simulink model "opti_debug"  (R2023a)
settings: Solver=FixedStepAuto  StartTime=0.0  StopTime=mdl.rt  RelTol=1e-3
values from neighbouring files (symbols this model uses):
  archived_Eul_XYZ = rst_Eul_XYZ.signals.values    [s4_run.m]    (also in step4_run_v1.m)
  archived_p_raw = rst_p_raw.signals.values    [s4_run.m]    (also in step4_run_v1.m)
  ctr = make_ext_tor_observer(rsim, mdl, ctr)    [s1_setup.m]    (also in setup_controller_with_functions.m = make_controller(); step1_setup.m; step1_setup_v1.m)
  ctr2 = ctr    [s1_setup.m]    (also in step1_setup.m; step1_setup_v1.m)
  lut = gen_lut    [s1_setup.m]    (also in thrust2voltage_lut_20230809.mat = ; thrust2voltage_lut_20230829.mat = )
  mdl = make_model(mdl,rsim)    [s1_setup.m]    (also in setup_controller_with_functions.m = make_model(flight_time); step1_setup.m; step1_setup_v1.m = make_model(flight_time,rsim))
  rbt = make_robot    [s1_setup.m]    (also in setup_controller_with_functions.m = make_robot(); step1_setup.m; step1_setup_v1.m)
  rbt2 = rbt    [s1_setup.m]    (also in step1_setup.m; step1_setup_v1.m)
  rsim = make_robot_simulation()    [setup_controller_with_functions.m]    (also in step1_setup_v1.m = make_simulation(rbt,mdl,rsim))
  sen = make_sensor(mdl,rsim)    [s1_setup.m]
  som = make_somersault(mdl, rsim)    [s1_setup.m]    (also in step1_setup.m)
  Time = logsout.LiveStreamSignals.getElement('voltage').Values.Time    [old_step3_run_controller_v3.m]    (also in post_identify_actuation_response.m = yout(:,1); post_thrust_torque_coefficients.m = yout(:,1))
  traj = make_trajectory(ctr, mdl, rsim)    [s1_setup.m]    (also in step1_setup.m)
undefined symbols (not defined in the file or in its folder): DiscIntNeverNeededParam, Discrete, Standard_Devices, UDP_Protocol
libraries: simulink x27, dspfdesign x12, robotcorelib x7, sldrtlib x7, slrealtimeloglib x1, shared6dof x1, dspsrcs4 x1, uavutilslib x1, ctrlSharedLib x1, dspmathops x1
(part 2 of 4)

== system opti_debug/Motor thrust to voltage mapping/back mapping from sat volt to torque-thrust ==
  sat_voltages : Inport
  Demux5 : Demux
  Digital Filter Design2 : dspfdesign/Digital Filter Design  mwdsp_browser_bugfix_var=off
  Mux10 : Mux
  Nemo Bee 1 : Lookup_n-D  NumberOfTableDimensions=1  BreakpointsForDimension1=lut.v4  Table=lut.T4  InternalRulePriority=Speed  RndMeth=Simplest
  Nemo Bee 2 : Lookup_n-D  NumberOfTableDimensions=1  BreakpointsForDimension1=lut.v1  Table=lut.T1  InternalRulePriority=Speed  RndMeth=Simplest
  Nemo Bee 3 : Lookup_n-D  NumberOfTableDimensions=1  BreakpointsForDimension1=lut.v3  Table=lut.T3  InternalRulePriority=Speed  RndMeth=Simplest
  Nemo Bee 4 : Lookup_n-D  NumberOfTableDimensions=1  BreakpointsForDimension1=lut.v2  Table=lut.T2  InternalRulePriority=Speed  RndMeth=Simplest
  Saturation{6..9} (4 alike) : Saturate  UpperLimit=1000  LowerLimit=0
  Scope : Scope  NumInputPorts=2
  Scope1 : Scope  Commented=on
  power_distribution_1 : MATLAB Function  TreatAsAtomicUnit=on
  torque_thrust : Outport
  wires:
  Saturation9/1 -> Mux10/4
  Saturation7/1 -> Mux10/2
  Nemo Bee 1/1 -> Saturation9/1
  Demux5/3 -> Nemo Bee 3/1
  Demux5/1 -> Nemo Bee 2/1
  Nemo Bee 2/1 -> Saturation6/1
  Demux5/4 -> Nemo Bee 1/1
  Saturation8/1 -> Mux10/3
  Nemo Bee 4/1 -> Saturation7/1
  Saturation6/1 -> Mux10/1
  Nemo Bee 3/1 -> Saturation8/1
  Demux5/2 -> Nemo Bee 4/1
  sat_voltages/1 -> Demux5/1
  power_distribution_1/1(torque_thrust) -> Scope1/1, torque_thrust/1
  Mux10/1 -> Digital Filter Design2/1, Scope/1  "sat motor thrust (mgf)"
  Digital Filter Design2/1 -> power_distribution_1/1(motor_thrust), Scope/2  "filtered mtor thrust (mgf)"

== system opti_debug/Motor thrust to voltage mapping/voltage safety (no imag & NaN) ==
  In1 : Inport
  Complex to Real-Imag{,1..3} (4 alike) : ComplexToRealImag
  Delay{,1..3} (4 alike) : Delay  DelayLength=1
  Demux : Demux
  IsNaN{,1..3} (4 alike) : RelationalOperator  Operator=isNaN  OutDataTypeStr=boolean  RndMeth=Simplest  InputSameDT=off
  Mux : Mux
  Switch{1..3,17} (4 alike) : Switch  Criteria=u2 > Threshold  SaturateOnIntegerOverflow=off  InputSameDT=off
  Terminator{,1..3} (4 alike) : Terminator
  Output : Outport
  wires:
  In1/1 -> Demux/1
  IsNaN/1 -> Switch17/2
  Switch17/1 -> Delay1/1, Complex to Real-Imag/1
  Complex to Real-Imag/2 -> Terminator/1
  Demux/1 -> Switch17/3, IsNaN/1
  Complex to Real-Imag1/2 -> Terminator1/1
  Complex to Real-Imag1/1 -> Mux/2
  IsNaN1/1 -> Switch1/2
  Switch1/1 -> Delay/1, Complex to Real-Imag1/1
  Demux/2 -> Switch1/3, IsNaN1/1
  Complex to Real-Imag2/2 -> Terminator2/1
  Complex to Real-Imag2/1 -> Mux/3
  IsNaN2/1 -> Switch2/2
  Switch2/1 -> Delay2/1, Complex to Real-Imag2/1
  Demux/3 -> Switch2/3, IsNaN2/1
  Complex to Real-Imag3/2 -> Terminator3/1
  Complex to Real-Imag3/1 -> Mux/4
  IsNaN3/1 -> Switch3/2
  Demux/4 -> IsNaN3/1, Switch3/3
  Switch3/1 -> Delay3/1, Complex to Real-Imag3/1
  Mux/1 -> Output/1
  Complex to Real-Imag/1 -> Mux/1
  Delay/1 -> Switch1/1
  Delay1/1 -> Switch17/1
  Delay2/1 -> Switch2/1
  Delay3/1 -> Switch3/1

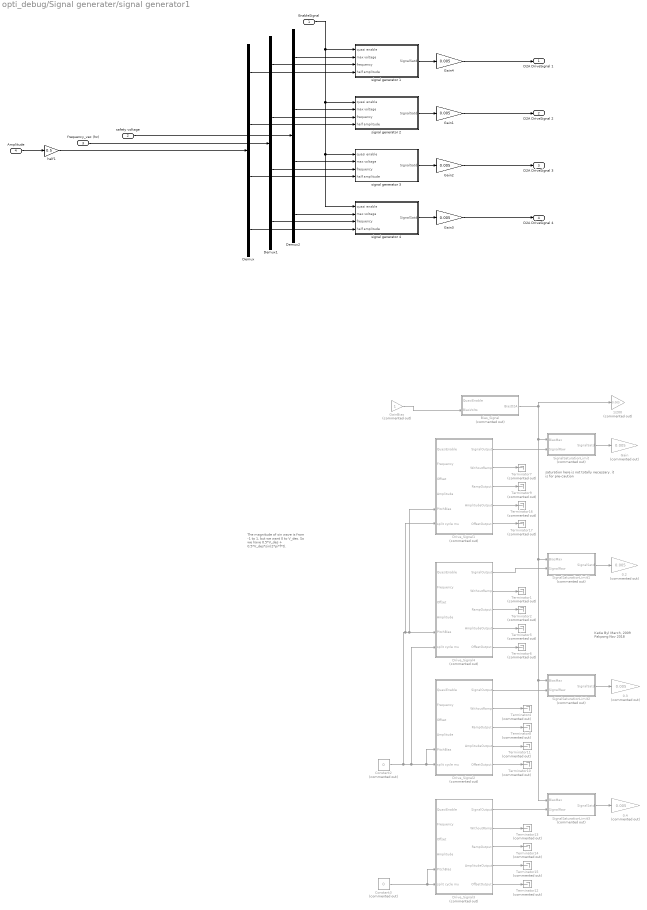
== system opti_debug/Signal generater/signal generator1 ==
  note: The magnitude of sin wave is from -1 to 1, but we want 0 to V_des. So we have 0.5*V_des + 0.5*V_des*sin(2*pi*f*t).
  note: Katie Byl
      | March, 2009
      |
      | Pakpong
      | Nov 2018
  note: saturation here is not totally necessary.
      | it is for pre-caution
  EnableSignal : Inport
  safety voltage : Inport  Port=2
  frequency_vec (hz) : Inport  Port=3
  Amplitude : Inport  Port=4
  0.2 : Gain  Commented=on  Gain=0.005
  0.3 : Gain  Commented=on  Gain=0.005
  0.4 : Gain  Commented=on  Gain=0.005
  1/200 : Gain  Commented=on  Gain=0.005
  Bias_Signal : Subsystem  Commented=on
  Constant2 : Constant  Commented=on  Value=0
  Constant3 : Constant  Commented=on  Value=0
  Demux : Demux
  Demux1 : Demux
  Demux2 : Demux
  Drive_Signal1 : Subsystem  Commented=on
  Drive_Signal2 : Subsystem  Commented=on
  Drive_Signal3 : Subsystem  Commented=on
  Drive_Signal4 : Subsystem  Commented=on
  Gain : Gain  Commented=on  Gain=0.005
  Gain{1..4} (4 alike) : Gain  Gain=0.005
  GainBias : Gain  Commented=on
  SignalSaturationLimit : Subsystem  Commented=on
  SignalSaturationLimit1 : Subsystem  Commented=on
  SignalSaturationLimit2 : Subsystem  Commented=on
  SignalSaturationLimit3 : Subsystem  Commented=on
  Terminator{1..2,4..17} (16 alike) : Terminator  Commented=on
  half1 : Gain  Gain=0.5
  signal generator 1 : Subsystem
  signal generator 2 : Subsystem
  signal generator 3 : Subsystem
  signal generator 4 : Subsystem
  D2A DriveSignal 1 : Outport
  D2A DriveSignal 2 : Outport  Port=2
  D2A DriveSignal 3 : Outport  Port=3
  D2A DriveSignal 4 : Outport  Port=4
  wires:
  Bias_Signal/1(BiasD2A) -> 1/200/1, SignalSaturationLimit3/1(BiasMax), SignalSaturationLimit2/1(BiasMax), SignalSaturationLimit1/1(BiasMax), SignalSaturationLimit/1(BiasMax)
  EnableSignal/1 -> signal generator 4/1(quasi enable), signal generator 3/1(quasi enable), signal generator 2/1(quasi enable), signal generator 1/1(quasi enable)
  SignalSaturationLimit/1(SignalSatd) -> Gain/1
  GainBias/1 -> Bias_Signal/2(BiasVolts)
  SignalSaturationLimit1/1(SignalSatd) -> 0.2/1
  Amplitude/1 -> half1/1
  Drive_Signal3/4(AmplitudeOutput) -> Terminator15/1
  Drive_Signal3/2(WithoutRamp) -> Terminator13/1
  Drive_Signal3/3(RampOutput) -> Terminator14/1
  Drive_Signal3/5(OffsetOutput) -> Terminator12/1
  Drive_Signal2/3(RampOutput) -> Terminator8/1
  Drive_Signal2/4(AmplitudeOutput) -> Terminator11/1
  Drive_Signal3/1(SignalOutput) -> SignalSaturationLimit3/2(SignalRaw)
  Drive_Signal2/5(OffsetOutput) -> Terminator10/1
  Drive_Signal2/2(WithoutRamp) -> Terminator4/1
  Demux/3 -> signal generator 3/4(half amplitude)
  Demux/4 -> signal generator 4/4(half amplitude)
  Constant2/1 -> Drive_Signal1/6(split cycle mu), Drive_Signal1/5(PitchBias), Drive_Signal4/5(PitchBias), Drive_Signal4/6(split cycle mu), Drive_Signal2/5(PitchBias), Drive_Signal2/6(split cycle mu)
  Constant3/1 -> Drive_Signal3/5(PitchBias), Drive_Signal3/6(split cycle mu)
  SignalSaturationLimit2/1(SignalSatd) -> 0.3/1
  SignalSaturationLimit3/1(SignalSatd) -> 0.4/1
  Drive_Signal2/1(SignalOutput) -> SignalSaturationLimit2/2(SignalRaw)
  half1/1 -> Demux/1
  frequency_vec (hz)/1 -> Demux1/1
  Demux1/1 -> signal generator 1/3(frequency)
  Demux1/2 -> signal generator 2/3(frequency)
  Demux1/3 -> signal generator 3/3(frequency)
  Demux1/4 -> signal generator 4/3(frequency)
  Drive_Signal4/1(SignalOutput) -> SignalSaturationLimit1/2(SignalRaw)
  Drive_Signal4/2(WithoutRamp) -> Terminator1/1
  Drive_Signal4/3(RampOutput) -> Terminator2/1
  Drive_Signal4/4(AmplitudeOutput) -> Terminator5/1
  Drive_Signal4/5(OffsetOutput) -> Terminator6/1
  Drive_Signal1/4(AmplitudeOutput) -> Terminator16/1
  Drive_Signal1/1(SignalOutput) -> SignalSaturationLimit/2(SignalRaw)
  Drive_Signal1/2(WithoutRamp) -> Terminator7/1
  Drive_Signal1/5(OffsetOutput) -> Terminator17/1
  Drive_Signal1/3(RampOutput) -> Terminator9/1
  Demux/1 -> signal generator 1/4(half amplitude)
  Demux/2 -> signal generator 2/4(half amplitude)
  signal generator 2/1(SignalSatd) -> Gain1/1
  signal generator 3/1(SignalSatd) -> Gain2/1
  signal generator 4/1(SignalSatd) -> Gain3/1
  signal generator 1/1(SignalSatd) -> Gain4/1
  Gain3/1 -> D2A DriveSignal 4/1
  Gain2/1 -> D2A DriveSignal 3/1
  Gain1/1 -> D2A DriveSignal 2/1
  Gain4/1 -> D2A DriveSignal 1/1
  safety voltage/1 -> Demux2/1
  Demux2/1 -> signal generator 1/2(max voltage)
  Demux2/2 -> signal generator 2/2(max voltage)
  Demux2/3 -> signal generator 3/2(max voltage)
  Demux2/4 -> signal generator 4/2(max voltage)

== system opti_debug/Signal generater/signal safety (no imag & NaN) ==
  In1 : Inport
  Complex to Real-Imag{,1..3} (4 alike) : ComplexToRealImag
  Constant{,1..3} (4 alike) : Constant  Value=0
  Demux : Demux
  IsNaN{,1..3} (4 alike) : RelationalOperator  Operator=isNaN  OutDataTypeStr=boolean  RndMeth=Simplest  InputSameDT=off
  Mux : Mux
  Switch{1..3,17} (4 alike) : Switch  Criteria=u2 > Threshold  SaturateOnIntegerOverflow=off  InputSameDT=off
  Terminator{,1..3} (4 alike) : Terminator
  Output : Outport
  wires:
  In1/1 -> Demux/1
  IsNaN/1 -> Switch17/2
  Constant/1 -> Switch17/1
  Switch17/1 -> Complex to Real-Imag/1
  Complex to Real-Imag/2 -> Terminator/1
  Demux/1 -> Switch17/3, IsNaN/1
  Complex to Real-Imag1/2 -> Terminator1/1
  Complex to Real-Imag1/1 -> Mux/2
  IsNaN1/1 -> Switch1/2
  Switch1/1 -> Complex to Real-Imag1/1
  Demux/2 -> Switch1/3, IsNaN1/1
  Constant1/1 -> Switch1/1
  Complex to Real-Imag2/2 -> Terminator2/1
  Complex to Real-Imag2/1 -> Mux/3
  IsNaN2/1 -> Switch2/2
  Switch2/1 -> Complex to Real-Imag2/1
  Demux/3 -> Switch2/3, IsNaN2/1
  Constant2/1 -> Switch2/1
  Complex to Real-Imag3/2 -> Terminator3/1
  Complex to Real-Imag3/1 -> Mux/4
  IsNaN3/1 -> Switch3/2
  Demux/4 -> IsNaN3/1, Switch3/3
  Switch3/1 -> Complex to Real-Imag3/1
  Constant3/1 -> Switch3/1
  Mux/1 -> Output/1
  Complex to Real-Imag/1 -> Mux/1

== system opti_debug/State filters/Acc through derivative ==
  Vicon_p_dot : Inport
  sim_p_dot : Inport  Port=2
  data ready : Inport  Port=3
  Add2 : Sum  Inputs=+-
  Constant3 : Constant  Value=rsim.en
  Delay1 : Delay  DelayLength=1  InitialCondition=zeros(3,1)
  Gain1 : Gain  Gain=400
  Subsystem1 : Subsystem
  Switch2 : Switch  Criteria=u2 > Threshold  SaturateOnIntegerOverflow=off  InputSameDT=off
  p_dotdot : Outport
  wires:
  Subsystem1/1(p_dotdot) -> Switch2/3
  sim_p_dot/1 -> Delay1/1, Add2/1
  Add2/1 -> Gain1/1
  Constant3/1 -> Switch2/2
  Delay1/1 -> Add2/2
  Vicon_p_dot/1 -> Subsystem1/1(p_dot)
  Switch2/1 -> p_dotdot/1  "p_dotdot"
  Gain1/1 -> Switch2/1
  data ready/1 -> Subsystem1/2(data ready)

== system opti_debug/State filters/IMU orientation ==
  sensor_Eul_XYZ : Inport
  Digital Filter Design1 : dspfdesign/Digital Filter Design  mwdsp_browser_bugfix_var=off
  Reshape2 : Reshape
  Subsystem2 : Subsystem
  Sensor_EulXYZ : Outport
  sensor_raw_omega : Outport  Port=2
  sensor_filt_omega : Outport  Port=3
  wires:
  sensor_Eul_XYZ/1 -> Subsystem2/1(euler_angles), Reshape2/1
  Digital Filter Design1/1 -> sensor_filt_omega/1  "sensor_filt_omega"
  Subsystem2/1(Omega) -> sensor_raw_omega/1, Digital Filter Design1/1  "sensor_raw_omega"
  Reshape2/1 -> Sensor_EulXYZ/1  "sensor_EulXYZ"

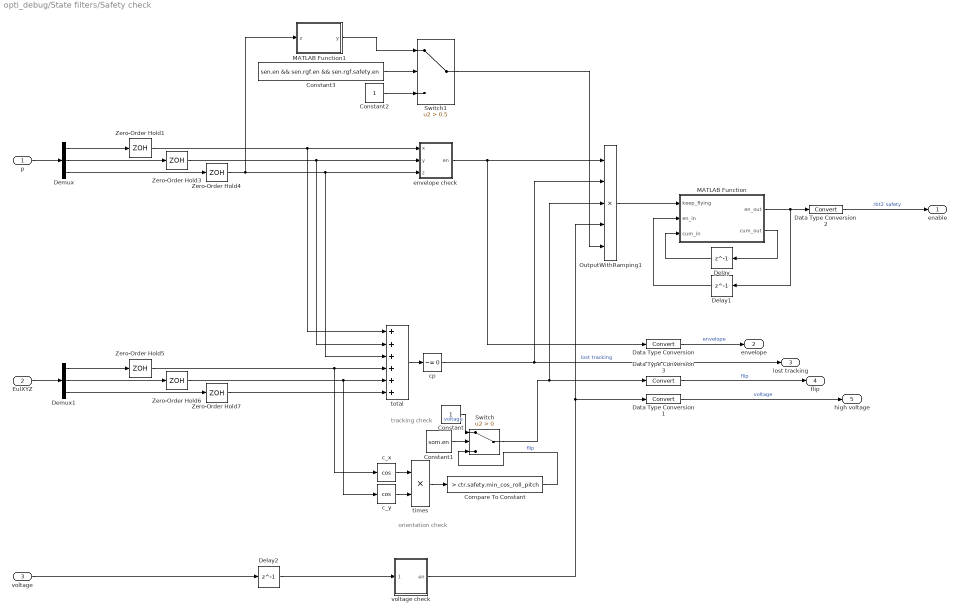
== system opti_debug/State filters/Safety check ==
  note: tracking check
  note: orientation check
  p : Inport
  EulXYZ : Inport  Port=2
  voltage : Inport  Port=3
  Compare To Constant : simulink/Logic and Bit Operations/Compare To Constant  relop=>  const=ctr.safety.min_cos_roll_pitch  OutDataTypeStr=uint8
  Constant : Constant
  Constant1 : Constant  Value=som.en
  Constant2 : Constant
  Constant3 : Constant  Value=sen.en && sen.rgf.en && sen.rgf.safety.en
  Data Type Conversion{,1..3} (4 alike) : DataTypeConversion  SaturateOnIntegerOverflow=off  RndMeth=Floor
  Delay : Delay  DelayLength=1
  Delay1 : Delay  DelayLength=1  InitialCondition=1
  Delay2 : Delay  DelayLength=1  InitialCondition=zeros(4,1)
  Demux : Demux  Outputs=3
  Demux1 : Demux  Outputs=3
  MATLAB Function : MATLAB Function  TreatAsAtomicUnit=on  SystemSampleTime=mdl.T
  MATLAB Function1 : MATLAB Function  TreatAsAtomicUnit=on
  OutputWithRamping1 : Product  Inputs=5  RndMeth=Zero
  Switch : Switch  Criteria=u2 > Threshold  SaturateOnIntegerOverflow=off  InputSameDT=off
  Switch1 : Switch  Criteria=u2 > Threshold  Threshold=0.5  SaturateOnIntegerOverflow=off  InputSameDT=off
  Zero-Order Hold{1,3..7} (6 alike) : ZeroOrderHold  SampleTime=mdl.T
  c_x : Trigonometry  Operator=cos
  c_y : Trigonometry  Operator=cos
  cp : simulink/Logic and Bit Operations/Compare To Zero  relop=~=  OutDataTypeStr=uint8
  envelope check : MATLAB Function  TreatAsAtomicUnit=on
  times : Product  RndMeth=Zero
  total : Sum  Inputs=++++++
  voltage check : MATLAB Function  TreatAsAtomicUnit=on
  enable : Outport
  envelope : Outport  Port=2
  lost tracking : Outport  Port=3
  flip : Outport  Port=4
  high voltage : Outport  Port=5
  wires:
  Zero-Order Hold3/1 -> envelope check/2(y), total/2
  cp/1 -> lost tracking/1, OutputWithRamping1/2  "lost tracking"
  Demux/3 -> Zero-Order Hold4/1
  times/1 -> Compare To Constant/1
  envelope check/1(en) -> Data Type Conversion/1, OutputWithRamping1/1
  Zero-Order Hold1/1 -> total/1, envelope check/1(x)
  Demux/2 -> Zero-Order Hold3/1
  OutputWithRamping1/1 -> MATLAB Function/1(keep_flying)
  Zero-Order Hold4/1 -> MATLAB Function1/1(z), total/3, envelope check/3(z)
  Demux1/2 -> Zero-Order Hold6/1
  MATLAB Function/2(cum_out) -> Delay/1
  Delay1/1 -> MATLAB Function/2(en_in)
  Data Type Conversion1/1 -> high voltage/1  "voltage"
  Data Type Conversion/1 -> envelope/1  "envelope"
  Delay2/1 -> voltage check/1(voltage)
  Switch/1 -> OutputWithRamping1/3, Data Type Conversion3/1
  total/1 -> cp/1
  Zero-Order Hold7/1 -> total/6
  Zero-Order Hold6/1 -> total/5, c_y/1
  voltage/1 -> Delay2/1
  Compare To Constant/1 -> Switch/3  "flip"
  MATLAB Function/1(en_out) -> Delay1/1, Data Type Conversion2/1
  Data Type Conversion2/1 -> enable/1  "rbt2 safety"
  Data Type Conversion3/1 -> flip/1  "flip"
  Constant1/1 -> Switch/2
  c_y/1 -> times/2
  Demux1/3 -> Zero-Order Hold7/1
  Delay/1 -> MATLAB Function/3(cum_in)
  voltage check/1(en) -> OutputWithRamping1/4, Data Type Conversion1/1
  Constant/1 -> Switch/1  "voltage"
  c_x/1 -> times/1
  Zero-Order Hold5/1 -> total/4, c_x/1
  p/1 -> Demux/1
  Demux/1 -> Zero-Order Hold1/1
  EulXYZ/1 -> Demux1/1
  Demux1/1 -> Zero-Order Hold5/1
  Constant2/1 -> Switch1/3
  Constant3/1 -> Switch1/2
  MATLAB Function1/1(y) -> Switch1/1
  Switch1/1 -> OutputWithRamping1/5

== system opti_debug/State filters/Velocity through derivative ==
  Vicon_p : Inport
  data ready : Inport  Port=2
  Add1 : Sum  Inputs=+-
  Constant2 : Constant  Value=rsim.en
  Delay : Delay  DelayLength=1  InitialCondition=zeros(3,1)
  Gain : Gain  Gain=400
  Subsystem4 : Subsystem
  Switch1 : Switch  Criteria=u2 > Threshold  SaturateOnIntegerOverflow=off  InputSameDT=off
  Vicon_p_dot : Outport
  sim_p_dot : Outport  Port=2
  wires:
  Delay/1 -> Add1/2
  Subsystem4/1(p dot) -> Switch1/3
  Vicon_p/1 -> Subsystem4/1(In1), Delay/1, Add1/1
  Constant2/1 -> Switch1/2
  Add1/1 -> Gain/1
  Switch1/1 -> Vicon_p_dot/1  "Vicon_p_dot"
  data ready/1 -> Subsystem4/2(data ready)
  Gain/1 -> sim_p_dot/1, Switch1/1  "sim_p_dot"

== system opti_debug/State filters/Vicon orientation ==
  Eul XYZ : Inport
  data_ready : Inport  Port=2
  Digital Filter Design2 : dspfdesign/Digital Filter Design  mwdsp_browser_bugfix_var=off
  Reshape1 : Reshape
  Subsystem5 : Subsystem
  Terminator8 : Terminator
  Terminator9 : Terminator
  Vicon_EulXYZ : Outport
  Vicon_raw_omega : Outport  Port=2
  Vicon_filt_omega : Outport  Port=3
  wires:
  Eul XYZ/1 -> Reshape1/1, Subsystem5/1(euler_angles)
  Reshape1/1 -> Vicon_EulXYZ/1  "Vicon_EulXYZ"
  Subsystem5/2(Rdot) -> Terminator9/1
  Subsystem5/3(Omega) -> Vicon_raw_omega/1, Digital Filter Design2/1  "Vicon_raw_omega"
  Subsystem5/1(R) -> Terminator8/1
  Digital Filter Design2/1 -> Vicon_filt_omega/1  "Vicon_filt_omega"
  data_ready/1 -> Subsystem5/2(data ready)

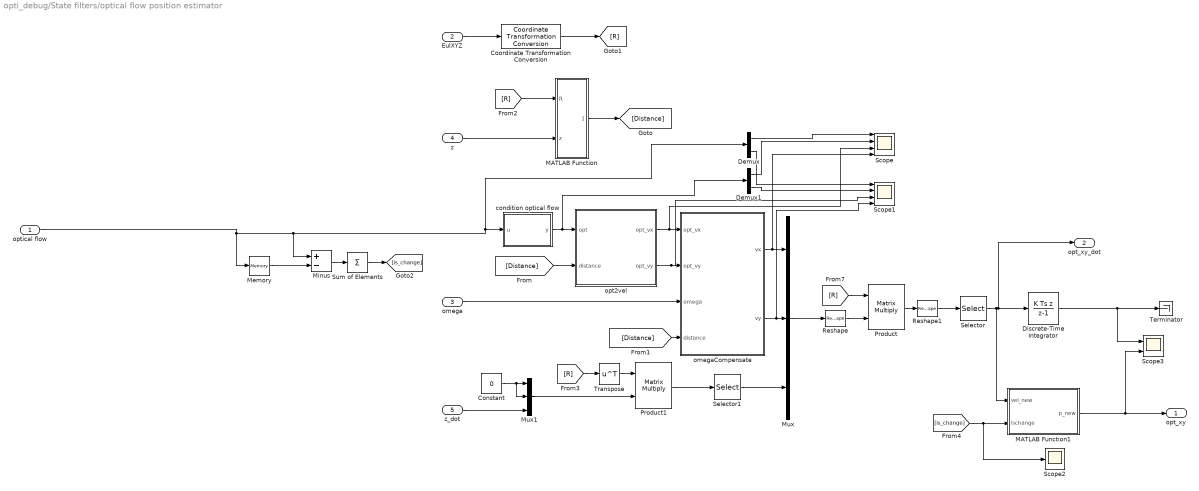
== system opti_debug/State filters/optical flow position estimator ==
  optical flow : Inport
  EulXYZ : Inport  Port=2
  omega : Inport  Port=3
  z : Inport  Port=4
  z_dot : Inport  Port=5
  Constant : Constant  Value=0
  Coordinate Transformation Conversion : robotcorelib/Coordinate Transformation Conversion  InputRepresentation=Euler Angles  InputEulerSequence=XYZ  ShowTrVecInputPort=on  OutputRepresentation=Rotation Matrix  OutputEulerSequence=ZYX  ShowTrVecOutputPort=on  SimulateUsing=Interpreted execution
  Demux : Demux  Outputs=2
  Demux1 : Demux  Outputs=2
  Discrete-Time Integrator : DiscreteIntegrator  IntegratorMethod=Integration: Backward Euler  InitialCondition=[0;0]  SampleTime=-1  ICPrevOutput=DiscIntNeverNeededParam  ICPrevScaledInput=DiscIntNeverNeededParam
  MATLAB Function : MATLAB Function  TreatAsAtomicUnit=on  SystemSampleTime=mdl.T_high
  MATLAB Function1 : MATLAB Function  TreatAsAtomicUnit=on
  Memory : Memory
  Minus : Sum  Inputs=+-
  Mux : Mux  Inputs=3
  Mux1 : Mux  Inputs=3
  Product : Product  Multiplication=Matrix(*)
  Product1 : Product  Multiplication=Matrix(*)
  Reshape : Reshape  OutputDimensionality=Column vector (2-D)
  Reshape1 : Reshape
  Scope : Scope  NumInputPorts=4
  Scope1 : Scope  NumInputPorts=4
  Scope2 : Scope
  Scope3 : Scope  NumInputPorts=2
  Selector : Selector  InputPortWidth=3  IndexOptions=Index vector (dialog)  Indices=[1 2 ]  OutputSizes=1
  Selector1 : Selector  InputPortWidth=3  IndexOptions=Index vector (dialog)  Indices=[3 ]  OutputSizes=1
  Sum of Elements : Sum  Inputs=+
  Terminator : Terminator
  Transpose : Math  Operator=transpose
  condition optical flow : MATLAB Function  TreatAsAtomicUnit=on
  omegaCompensate : MATLAB Function  TreatAsAtomicUnit=on
  opt2vel : MATLAB Function  TreatAsAtomicUnit=on
  opt_xy : Outport
  opt_xy_dot : Outport  Port=2
  wires:
  EulXYZ/1 -> Coordinate Transformation Conversion/1
  z/1 -> MATLAB Function/2(z)
  MATLAB Function/1(distance) -> [Distance]
  [Distance] -> opt2vel/2(distance)
  opt2vel/1(opt_vx) -> Scope/3, omegaCompensate/1(opt_vx)
  opt2vel/2(opt_vy) -> Scope1/3, omegaCompensate/2(opt_vy)
  [Distance] -> omegaCompensate/4(distance)
  omega/1 -> omegaCompensate/3(omega)
  Coordinate Transformation Conversion/1 -> [R]
  [R] -> MATLAB Function/1(R)
  [R] -> Product/1
  Reshape/1 -> Product/2
  Mux/1 -> Reshape/1
  omegaCompensate/1(vx) -> Scope/4, Mux/1
  omegaCompensate/2(vy) -> Scope1/4, Mux/2
  Product/1 -> Reshape1/1
  Reshape1/1 -> Selector/1
  [R] -> Transpose/1
  Transpose/1 -> Product1/1
  Product1/1 -> Selector1/1
  Constant/1 -> Mux1/2, Mux1/1
  z_dot/1 -> Mux1/3
  Mux1/1 -> Product1/2
  Selector1/1 -> Mux/3
  Selector/1 -> MATLAB Function1/1(vel_new), opt_xy_dot/1, Discrete-Time Integrator/1
  condition optical flow/1(y) -> Demux1/1, opt2vel/1(opt)
  optical flow/1 -> Memory/1, Minus/1, Demux/1, condition optical flow/1(u)
  Demux/1 -> Scope/1
  Demux1/1 -> Scope/2
  Demux/2 -> Scope1/1
  Demux1/2 -> Scope1/2
  Memory/1 -> Minus/2
  Minus/1 -> Sum of Elements/1
  [is_change] -> Scope2/1, MATLAB Function1/2(ischange)
  Discrete-Time Integrator/1 -> Scope3/1, Terminator/1
  MATLAB Function1/1(p_new) -> Scope3/2, opt_xy/1
  Sum of Elements/1 -> [is_change]

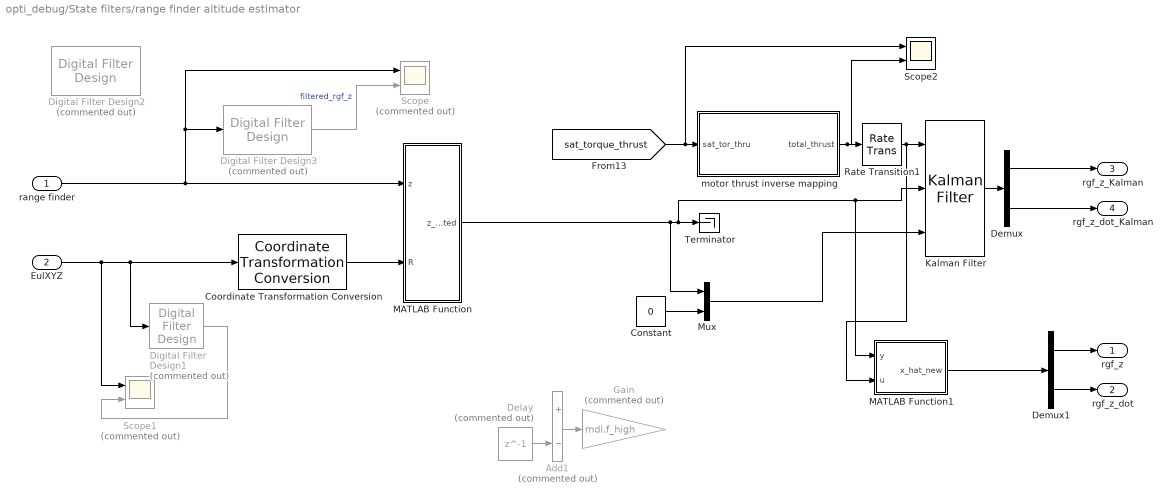
== system opti_debug/State filters/range finder altitude estimator ==
  range finder : Inport
  EulXYZ : Inport  Port=2
  Add1 : Sum  Commented=on  Inputs=+-
  Constant : Constant  Value=0
  Coordinate Transformation Conversion : robotcorelib/Coordinate Transformation Conversion  InputRepresentation=Euler Angles  InputEulerSequence=XYZ  ShowTrVecInputPort=on  OutputRepresentation=Rotation Matrix  OutputEulerSequence=ZYX  ShowTrVecOutputPort=on  SimulateUsing=Interpreted execution
  Delay : Delay  Commented=on  DelayLength=1  InitialCondition=0
  Demux : Demux  Outputs=2
  Demux1 : Demux  Outputs=2
  Digital Filter Design1 : dspfdesign/Digital Filter Design  Commented=on  mwdsp_browser_bugfix_var=off
  Digital Filter Design2 : dspfdesign/Digital Filter Design  Commented=on  mwdsp_browser_bugfix_var=off
  Digital Filter Design3 : dspfdesign/Digital Filter Design  Commented=on  mwdsp_browser_bugfix_var=off
  Gain : Gain  Commented=on  Gain=mdl.f_high
  Kalman Filter : ctrlSharedLib/Kalman Filter  TimeDomain=Discrete-Time  UseCurrentEstimator=on  ModelSource=Individual A, B, C, D matrices  ModelSourceVariable=ss(0.95,1,1,0,1)  A=[0,1;0,0]*mdl.T_high+eye(2)  B=[0;1/rbt.m]*mdl.T_high  C=[1,0]  D=0  NumberOfStates=1  NumberOfInputs=1  NumberOfOutputs=1  InitialEstimateSource=Input port  X0=0  P0=10  UseK=off  UseGH=on  NumberOfProcessNoiseInputs=1  G=[0;1/rbt.m]*mdl.T_high  TimeInvariantG=on  H=0  TimeInvariantH=on  Q=1e-7  TimeInvariantQ=on  R=5e-5  TimeInvariantR=on  N=0  TimeInvariantN=on  AddInputPort=on  AddEnablePort=off  OutputEstimatedY=off  OutputP=off  Ts=mdl.T_high
  MATLAB Function : MATLAB Function  TreatAsAtomicUnit=on  SystemSampleTime=mdl.T_high
  MATLAB Function1 : MATLAB Function  TreatAsAtomicUnit=on
  Mux : Mux  Inputs=2
  Rate Transition1 : RateTransition  OutPortSampleTime=mdl.T_high
  Scope : Scope  Commented=on  NumInputPorts=2
  Scope1 : Scope  Commented=on  NumInputPorts=2
  Scope2 : Scope  NumInputPorts=2
  Terminator : Terminator
  "motor thrust inverse mapping " : MATLAB Function  TreatAsAtomicUnit=on
  rgf_z : Outport
  rgf_z_dot : Outport  Port=2
  rgf_z_Kalman : Outport  Port=3
  rgf_z_dot_Kalman : Outport  Port=4
  wires:
  range finder/1 -> Digital Filter Design3/1, Scope/1, MATLAB Function/1(z)
  Digital Filter Design3/1 -> Scope/2  "filtered_rgf_z"
  EulXYZ/1 -> Coordinate Transformation Conversion/1, Digital Filter Design1/1, Scope1/1
  Coordinate Transformation Conversion/1 -> MATLAB Function/2(R)
  Add1/1 -> Gain/1
  Delay/1 -> Add1/2
  Digital Filter Design1/1 -> Scope1/2
  MATLAB Function/1(z_compensated) -> Mux/1, MATLAB Function1/1(y), Kalman Filter/2, Terminator/1
  Kalman Filter/1 -> Demux/1
  Demux/1 -> rgf_z_Kalman/1
  Demux/2 -> rgf_z_dot_Kalman/1
  [sat_torque_thrust] -> Scope2/1, "motor thrust inverse mapping "/1(sat_tor_thru)
  "motor thrust inverse mapping "/1(total_thrust) -> Scope2/2, Rate Transition1/1
  Rate Transition1/1 -> Kalman Filter/1, MATLAB Function1/2(u)
  Constant/1 -> Mux/2
  Mux/1 -> Kalman Filter/3
  MATLAB Function1/1(x_hat_new) -> Demux1/1
  Demux1/1 -> rgf_z/1
  Demux1/2 -> rgf_z_dot/1

== system opti_debug/UDP send to Arduino/UDP send to Arduino DAC ==
  note: Aptinex DAC 20230818
  DAC1 : Inport
  DAC2 : Inport  Port=2
  DAC3 : Inport  Port=3
  DAC4 : Inport  Port=4
  DO2 : Inport  Port=5  OutDataTypeStr=boolean
  Bit Set : simulink/Logic and Bit Operations/Bit Set  iBit=12
  Demux : Demux
  Gain{,1..3} (4 alike) : Gain  Gain=4095/10  OutDataTypeStr=uint16
  Mux : Mux
  Mux1 : Mux
  Saturation : Saturate  UpperLimit=10  LowerLimit=0
  Switch : Switch  Criteria=u2 ~= 0  OutDataTypeStr=uint16  SaturateOnIntegerOverflow=off  InputSameDT=off
  Output : Outport
  wires:
  Gain3/1 -> Mux1/4  "UDP uint16 4"
  Gain1/1 -> Mux1/2  "UDP uint16 2"
  Gain/1 -> Bit Set/1, Switch/3  "UDP uint16 1"
  Gain2/1 -> Mux1/3  "UDP uint16 3"
  DO2/1 -> Switch/2
  Bit Set/1 -> Switch/1
  Mux1/1 -> Output/1
  Switch/1 -> Mux1/1
  Demux/1 -> Gain/1
  Demux/2 -> Gain1/1
  Demux/3 -> Gain2/1
  Demux/4 -> Gain3/1
  DAC1/1 -> Mux/1  "DAC voltage 1"
  DAC2/1 -> Mux/2  "DAC voltage 2"
  DAC3/1 -> Mux/3  "DAC voltage 3"
  DAC4/1 -> Mux/4  "DAC voltage 4"
  Mux/1 -> Saturation/1
  Saturation/1 -> Demux/1

== system opti_debug/Control scheme/attitude and thrust controller/Subsystem ==
  att_e : Inport
  alt_e : Inport  Port=2
  Delay2 : Delay  DelayLength=1  InitialCondition=zeros(4,1)
  Digital Clock : DigitalClock  SampleTime=mdl.T
  Discrete-Time Integrator : DiscreteIntegrator  InitialCondition=zeros(4,1)  SampleTime=mdl.T  LimitOutput=on  UpperSaturationLimit=ctr.integral.lim.upper  LowerSaturationLimit=ctr.integral.lim.lower  ICPrevOutput=DiscIntNeverNeededParam  ICPrevScaledInput=DiscIntNeverNeededParam
  Gain : Gain  Gain=ctr.gain.ati
  Gain1 : Gain  Gain=ctr.gain.ali
  MATLAB Function : MATLAB Function  TreatAsAtomicUnit=on
  Mux : Mux  Inputs=2
  Product : Product
  Selector : Selector  InputPortWidth=4  IndexOptions=Index vector (dialog)  Indices=[1 2 3]  OutputSizes=1
  Selector1 : Selector  InputPortWidth=4  IndexOptions=Index vector (dialog)  Indices=[4]  OutputSizes=1
  int thrust : Scope
  int torque : Scope
  Out1 : Outport
  wires:
  Digital Clock/1 -> MATLAB Function/1(time)
  MATLAB Function/1(en_int) -> Product/1
  Mux/1 -> Product/2
  Discrete-Time Integrator/1 -> Delay2/1
  Selector1/1 -> int thrust/1  "int thrust acc"
  Delay2/1 -> Selector1/1, Selector/1, Out1/1
  Gain/1 -> Mux/1
  att_e/1 -> Gain/1
  Product/1 -> Discrete-Time Integrator/1
  Selector/1 -> int torque/1  "int torque"
  Gain1/1 -> Mux/2
  alt_e/1 -> Gain1/1

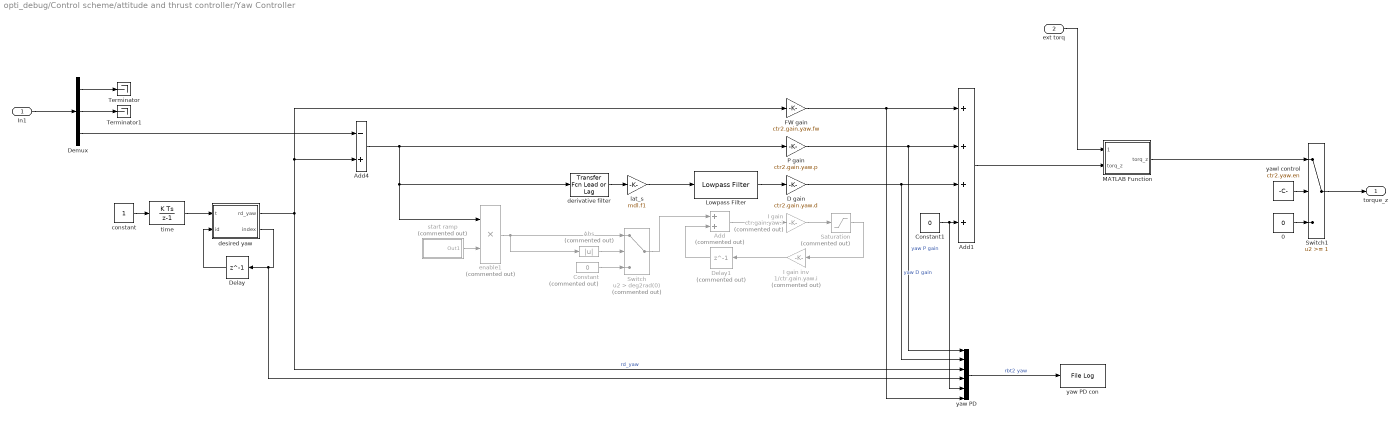
== system opti_debug/Control scheme/attitude and thrust controller/Yaw Controller ==
  In1 : Inport
  ext torq : Inport  Port=2
  0 : Constant  Value=0  SampleTime=-1
  Abs : Abs  Commented=on  SaturateOnIntegerOverflow=off
  Add : Sum  Commented=on
  Add1 : Sum  Inputs=++++
  Add4 : Sum  Inputs=-+
  Constant : Constant  Commented=on  Value=0
  Constant1 : Constant  Value=0  SampleTime=-1
  D gain : Gain  Gain=ctr2.gain.yaw.d
  Delay : Delay  DelayLength=1  InitialCondition=1
  Delay1 : Delay  Commented=on  DelayLength=1
  Demux : Demux  Outputs=3
  FW gain : Gain  Gain=ctr2.gain.yaw.fw
  I gain : Gain  Commented=on  Gain=ctr.gain.yaw.i
  I gain inv : Gain  Commented=on  Gain=1/ctr.gain.yaw.i
  Lowpass Filter : dspfdesign/Lowpass Filter  FilterType=FIR  DesignForMinimumOrder=on  FilterOrder=2000  PassbandFrequency=7  StopbandFrequency=90  PassbandRipple=0.5  StopbandAttenuation=75  SampleRateMode=Specify on dialog  SampleRate=10000  SimulateUsing=Interpreted execution  roundingMode=Floor  coeffsDataTypeStr=fixdt(1,16)
  MATLAB Function : MATLAB Function  TreatAsAtomicUnit=on
  P gain : Gain  Gain=ctr2.gain.yaw.p
  Saturation : Saturate  Commented=on  UpperLimit=ctr.integral.yaw.upper  LowerLimit=ctr.integral.yaw.lower
  Switch : Switch  Commented=on  Criteria=u2 > Threshold  Threshold=deg2rad(0)  SaturateOnIntegerOverflow=off  InputSameDT=off
  Switch1 : Switch  Threshold=1  SaturateOnIntegerOverflow=off  InputSameDT=off
  Terminator : Terminator
  Terminator1 : Terminator
  constant : Constant
  derivative filter : simulink/Discrete/Transfer Fcn Lead or Lag  PoleZ=mdl.zf1  ZeroZ=1  ICPrevOutput=0.0  ICPrevInput=0.0  DoSatur=off
  desired yaw : MATLAB Function  TreatAsAtomicUnit=on
  enable1 : Product  Commented=on  Inputs=**
  lat_s : Gain  Gain=mdl.f1
  start ramp : Subsystem  Commented=on
  time : DiscreteIntegrator  gainval=1  SampleTime=-1  UpperSaturationLimit=1  LowerSaturationLimit=0  ICPrevOutput=DiscIntNeverNeededParam  ICPrevScaledInput=DiscIntNeverNeededParam
  yaw PD : Mux  Inputs=6
  yaw PD con : slrealtimeloglib/File Log  decimation=1  inputProcessing=Elements as channels (sample based)
  yawl control : Constant  Value=ctr2.yaw.en
  torque_z : Outport
  wires:
  Demux/1 -> Terminator/1
  Demux/2 -> Terminator1/1
  Demux/3 -> Add4/1
  0/1 -> Switch1/3
  yawl control/1 -> Switch1/2
  In1/1 -> Demux/1
  Add4/1 -> P gain/1, enable1/1, derivative filter/1
  Switch1/1 -> torque_z/1
  derivative filter/1 -> lat_s/1
  Add1/1 -> MATLAB Function/2("torq_z ")
  P gain/1 -> yaw PD/1, Add1/2  "yaw P gain"
  D gain/1 -> yaw PD/2, Add1/3  "yaw D gain"
  yaw PD/1 -> yaw PD con/1  "rbt2 yaw"
  Lowpass Filter/1 -> D gain/1
  lat_s/1 -> Lowpass Filter/1
  constant/1 -> time/1
  time/1 -> desired yaw/1(t)
  desired yaw/1(rd_yaw) -> FW gain/1, Add4/2, yaw PD/3  "rd_yaw"
  desired yaw/2(index) -> yaw PD/4, Delay/1
  Delay/1 -> desired yaw/2(id)
  Saturation/1 -> I gain inv/1
  I gain/1 -> Saturation/1
  enable1/1 -> Switch/1, Abs/1
  Delay1/1 -> Add/2
  Add/1 -> I gain/1
  I gain inv/1 -> Delay1/1
  start ramp/1(Out1) -> enable1/2
  Constant/1 -> Switch/3
  Switch/1 -> Add/1
  Abs/1 -> Switch/2
  FW gain/1 -> yaw PD/6, Add1/1
  Constant1/1 -> yaw PD/5, Add1/4
  MATLAB Function/1(torq_z) -> Switch1/1
  ext torq/1 -> MATLAB Function/1(torq_ext)

== system opti_debug/Control scheme/attitude and thrust controller/time ==
  constant : Constant
  time : DiscreteIntegrator  gainval=1  SampleTime=-1  UpperSaturationLimit=1  LowerSaturationLimit=0  ICPrevOutput=DiscIntNeverNeededParam  ICPrevScaledInput=DiscIntNeverNeededParam
  real times : Outport
  wires:
  constant/1 -> time/1
  time/1 -> real times/1

== system opti_debug/Control scheme/observer/Rotaion ==
  Euler : Inport
  Rotation Matrix : MATLAB Function  TreatAsAtomicUnit=on
  Rotation Matrix1 : MATLAB Function  TreatAsAtomicUnit=on
  filtered derivative : Subsystem
  R : Outport
  Rdot : Outport  Port=2
  Omega : Outport  Port=3
  wires:
  Rotation Matrix/1(R) -> filtered derivative/1(In1), Rotation Matrix1/1(R), R/1
  Euler/1 -> Rotation Matrix/1(euler_angles)
  filtered derivative/1(Out1) -> Rotation Matrix1/2(Rdot), Rdot/1
  Rotation Matrix1/1(w) -> Omega/1

== system opti_debug/Control scheme/observer/lateral observer ==
  XYZ : Inport
  derivative filter : simulink/Discrete/Transfer Fcn Lead or Lag  PoleZ=mdl.zf1  ZeroZ=1  ICPrevOutput=0.0  ICPrevInput=0.0  DoSatur=off
  derivative filter1 : simulink/Discrete/Transfer Fcn Lead or Lag  PoleZ=mdl.zf2  ZeroZ=1  ICPrevOutput=0.0  ICPrevInput=0.0  DoSatur=off
  derivative filter2 : simulink/Discrete/Transfer Fcn Lead or Lag  PoleZ=mdl.zf2  ZeroZ=1  ICPrevOutput=0.0  ICPrevInput=0.0  DoSatur=off
  lat_s : Gain  Gain=mdl.f1
  lat_s2 : Gain  Gain=mdl.f2
  lat_s2_ : Gain  Gain=mdl.f2
  saturation : Subsystem
  r : Outport
  r_dot : Outport  Port=2
  r_dotdot : Outport  Port=3
  wires:
  derivative filter1/1 -> derivative filter2/1
  derivative filter/1 -> lat_s/1
  XYZ/1 -> derivative filter/1, derivative filter1/1, r/1
  derivative filter2/1 -> lat_s2/1
  lat_s/1 -> r_dot/1
  lat_s2/1 -> lat_s2_/1
  lat_s2_/1 -> saturation/1(In1)
  saturation/1(Out1) -> r_dotdot/1

== system opti_debug/Motor thrust to voltage mapping/Subsystem/time ==
  constant : Constant
  time : DiscreteIntegrator  gainval=1  SampleTime=-1  UpperSaturationLimit=1  LowerSaturationLimit=0  ICPrevOutput=DiscIntNeverNeededParam  ICPrevScaledInput=DiscIntNeverNeededParam
  real times : Outport
  wires:
  constant/1 -> time/1
  time/1 -> real times/1

== system opti_debug/Signal generater/signal generator1/Bias_Signal ==
  note: time constant = 0.002sec
  QuasiEnable : Inport
  BiasVolts : Inport  Port=2
  AveragedBias : Subsystem
  PreGain : Gain
  Product : Product  RndMeth=Zero
  SIgnalForRamp_binary : Subsystem
  SaturatingRamp : DiscreteIntegrator  gainval=100  SampleTime=-1  LimitOutput=on  UpperSaturationLimit=1  LowerSaturationLimit=0  ICPrevOutput=DiscIntNeverNeededParam  ICPrevScaledInput=DiscIntNeverNeededParam
  BiasD2A : Outport
  wires:
  PreGain/1 -> BiasD2A/1
  BiasVolts/1 -> AveragedBias/1(In1)
  QuasiEnable/1 -> SIgnalForRamp_binary/1(In1)
  SIgnalForRamp_binary/1(Out1) -> SaturatingRamp/1
  SaturatingRamp/1 -> Product/1
  AveragedBias/1(Out1) -> Product/2
  Product/1 -> PreGain/1

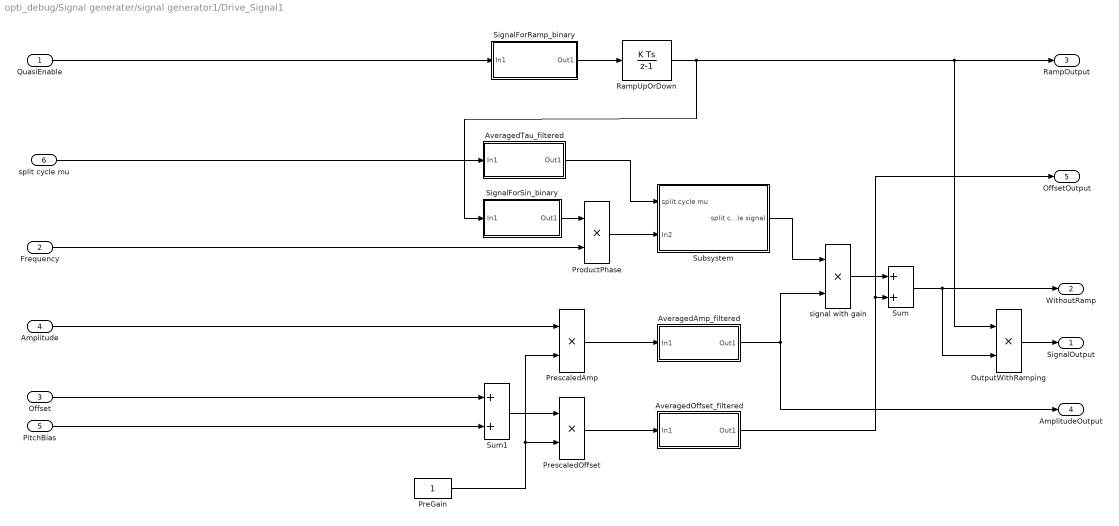
== system opti_debug/Signal generater/signal generator1/Drive_Signal1 ==
  QuasiEnable : Inport
  Frequency : Inport  Port=2
  Offset : Inport  Port=3
  Amplitude : Inport  Port=4
  PitchBias : Inport  Port=5
  split cycle mu : Inport  Port=6
  AveragedAmp_filtered : Subsystem
  AveragedOffset_filtered : Subsystem
  AveragedTau_filtered : Subsystem
  OutputWithRamping : Product  RndMeth=Zero
  PreGain : Constant
  PrescaledAmp : Product  RndMeth=Zero
  PrescaledOffset : Product  RndMeth=Zero
  ProductPhase : Product  RndMeth=Zero
  RampUpOrDown : DiscreteIntegrator  gainval=100  SampleTime=-1  LimitOutput=on  UpperSaturationLimit=1  LowerSaturationLimit=0  ICPrevOutput=DiscIntNeverNeededParam  ICPrevScaledInput=DiscIntNeverNeededParam
  SignalForRamp_binary : Subsystem
  SignalForSin_binary : Subsystem
  Subsystem : Subsystem
  Sum : Sum
  Sum1 : Sum
  signal with gain : Product  RndMeth=Zero
  SignalOutput : Outport
  WithoutRamp : Outport  Port=2
  RampOutput : Outport  Port=3
  AmplitudeOutput : Outport  Port=4
  OffsetOutput : Outport  Port=5
  wires:
  PrescaledAmp/1 -> AveragedAmp_filtered/1(In1)
  Sum/1 -> OutputWithRamping/2, WithoutRamp/1
  RampUpOrDown/1 -> RampOutput/1, OutputWithRamping/1, SignalForSin_binary/1(In1)
  QuasiEnable/1 -> SignalForRamp_binary/1(In1)
  SignalForRamp_binary/1(Out1) -> RampUpOrDown/1
  Amplitude/1 -> PrescaledAmp/1
  signal with gain/1 -> Sum/1
  Frequency/1 -> ProductPhase/2
  SignalForSin_binary/1(Out1) -> ProductPhase/1
  ProductPhase/1 -> Subsystem/2(In2)
  AveragedOffset_filtered/1(Out1) -> Sum/2, OffsetOutput/1
  PrescaledOffset/1 -> AveragedOffset_filtered/1(In1)
  PreGain/1 -> PrescaledAmp/2, PrescaledOffset/2
  OutputWithRamping/1 -> SignalOutput/1
  AveragedAmp_filtered/1(Out1) -> signal with gain/2, AmplitudeOutput/1
  Sum1/1 -> PrescaledOffset/1
  Offset/1 -> Sum1/1
  PitchBias/1 -> Sum1/2
  AveragedTau_filtered/1(Out1) -> Subsystem/1(split cycle mu)
  split cycle mu/1 -> AveragedTau_filtered/1(In1)
  Subsystem/1(split cycle signal) -> signal with gain/1

== system opti_debug/Signal generater/signal generator1/Drive_Signal2 ==
  QuasiEnable : Inport
  Frequency : Inport  Port=2
  Offset : Inport  Port=3
  Amplitude : Inport  Port=4
  PitchBias : Inport  Port=5
  split cycle mu : Inport  Port=6
  AveragedAmp_filtered : Subsystem  Commented=through
  AveragedOffset_filtered : Subsystem  Commented=through
  AveragedTau_filtered : Subsystem
  OutputWithRamping : Product  RndMeth=Zero
  PreGain : Constant
  PrescaledAmp : Product  RndMeth=Zero
  PrescaledOffset : Product  RndMeth=Zero
  ProductPhase : Product  RndMeth=Zero
  RampUpOrDown : DiscreteIntegrator  gainval=100  SampleTime=-1  LimitOutput=on  UpperSaturationLimit=1  LowerSaturationLimit=0  ICPrevOutput=DiscIntNeverNeededParam  ICPrevScaledInput=DiscIntNeverNeededParam
  SignalForRamp_binary : Subsystem
  SignalForSin_binary : Subsystem
  Subsystem : Subsystem
  Sum : Sum
  Sum1 : Sum
  signal with gain : Product  RndMeth=Zero
  SignalOutput : Outport
  WithoutRamp : Outport  Port=2
  RampOutput : Outport  Port=3
  AmplitudeOutput : Outport  Port=4
  OffsetOutput : Outport  Port=5
  wires:
  PrescaledAmp/1 -> AveragedAmp_filtered/1(In1)
  Sum/1 -> OutputWithRamping/2, WithoutRamp/1
  RampUpOrDown/1 -> RampOutput/1, OutputWithRamping/1, SignalForSin_binary/1(In1)
  QuasiEnable/1 -> SignalForRamp_binary/1(In1)
  SignalForRamp_binary/1(Out1) -> RampUpOrDown/1
  Amplitude/1 -> PrescaledAmp/1
  signal with gain/1 -> Sum/1
  Frequency/1 -> ProductPhase/2
  SignalForSin_binary/1(Out1) -> ProductPhase/1
  ProductPhase/1 -> Subsystem/2(In2)
  AveragedOffset_filtered/1(Out1) -> Sum/2, OffsetOutput/1
  PrescaledOffset/1 -> AveragedOffset_filtered/1(In1)
  PreGain/1 -> PrescaledAmp/2, PrescaledOffset/2
  OutputWithRamping/1 -> SignalOutput/1
  AveragedAmp_filtered/1(Out1) -> signal with gain/2, AmplitudeOutput/1
  Sum1/1 -> PrescaledOffset/1
  Offset/1 -> Sum1/1
  PitchBias/1 -> Sum1/2
  AveragedTau_filtered/1(Out1) -> Subsystem/1(split cycle mu)
  split cycle mu/1 -> AveragedTau_filtered/1(In1)
  Subsystem/1(split cycle signal) -> signal with gain/1

== system opti_debug/Signal generater/signal generator1/Drive_Signal3 ==
  QuasiEnable : Inport
  Frequency : Inport  Port=2
  Offset : Inport  Port=3
  Amplitude : Inport  Port=4
  PitchBias : Inport  Port=5
  split cycle mu : Inport  Port=6
  AveragedAmp_filtered : Subsystem  Commented=through
  AveragedOffset_filtered : Subsystem  Commented=through
  AveragedTau_filtered : Subsystem
  OutputWithRamping : Product  RndMeth=Zero
  PreGain : Constant
  PrescaledAmp : Product  RndMeth=Zero
  PrescaledOffset : Product  RndMeth=Zero
  ProductPhase : Product  RndMeth=Zero
  RampUpOrDown : DiscreteIntegrator  gainval=100  SampleTime=-1  LimitOutput=on  UpperSaturationLimit=1  LowerSaturationLimit=0  ICPrevOutput=DiscIntNeverNeededParam  ICPrevScaledInput=DiscIntNeverNeededParam
  SignalForRamp_binary : Subsystem
  SignalForSin_binary : Subsystem
  Subsystem : Subsystem
  Sum : Sum
  Sum1 : Sum
  signal with gain : Product  RndMeth=Zero
  SignalOutput : Outport
  WithoutRamp : Outport  Port=2
  RampOutput : Outport  Port=3
  AmplitudeOutput : Outport  Port=4
  OffsetOutput : Outport  Port=5
  wires:
  PrescaledAmp/1 -> AveragedAmp_filtered/1(In1)
  Sum/1 -> OutputWithRamping/2, WithoutRamp/1
  RampUpOrDown/1 -> RampOutput/1, OutputWithRamping/1, SignalForSin_binary/1(In1)
  QuasiEnable/1 -> SignalForRamp_binary/1(In1)
  SignalForRamp_binary/1(Out1) -> RampUpOrDown/1
  Amplitude/1 -> PrescaledAmp/1
  signal with gain/1 -> Sum/1
  Frequency/1 -> ProductPhase/2
  SignalForSin_binary/1(Out1) -> ProductPhase/1
  ProductPhase/1 -> Subsystem/2(In2)
  AveragedOffset_filtered/1(Out1) -> Sum/2, OffsetOutput/1
  PrescaledOffset/1 -> AveragedOffset_filtered/1(In1)
  PreGain/1 -> PrescaledAmp/2, PrescaledOffset/2
  OutputWithRamping/1 -> SignalOutput/1
  AveragedAmp_filtered/1(Out1) -> signal with gain/2, AmplitudeOutput/1
  Sum1/1 -> PrescaledOffset/1
  Offset/1 -> Sum1/1
  PitchBias/1 -> Sum1/2
  AveragedTau_filtered/1(Out1) -> Subsystem/1(split cycle mu)
  split cycle mu/1 -> AveragedTau_filtered/1(In1)
  Subsystem/1(split cycle signal) -> signal with gain/1

== system opti_debug/Signal generater/signal generator1/Drive_Signal4 ==
  QuasiEnable : Inport
  Frequency : Inport  Port=2
  Offset : Inport  Port=3
  Amplitude : Inport  Port=4
  PitchBias : Inport  Port=5
  split cycle mu : Inport  Port=6
  AveragedAmp_filtered : Subsystem
  AveragedOffset_filtered : Subsystem
  AveragedTau_filtered : Subsystem
  OutputWithRamping : Product  RndMeth=Zero
  PreGain : Constant
  PrescaledAmp : Product  RndMeth=Zero
  PrescaledOffset : Product  RndMeth=Zero
  ProductPhase : Product  RndMeth=Zero
  RampUpOrDown : DiscreteIntegrator  gainval=100  SampleTime=-1  LimitOutput=on  UpperSaturationLimit=1  LowerSaturationLimit=0  ICPrevOutput=DiscIntNeverNeededParam  ICPrevScaledInput=DiscIntNeverNeededParam
  SignalForRamp_binary : Subsystem
  SignalForSin_binary : Subsystem
  Subsystem : Subsystem
  Sum : Sum
  Sum1 : Sum
  signal with gain : Product  RndMeth=Zero
  SignalOutput : Outport
  WithoutRamp : Outport  Port=2
  RampOutput : Outport  Port=3
  AmplitudeOutput : Outport  Port=4
  OffsetOutput : Outport  Port=5
  wires:
  PrescaledAmp/1 -> AveragedAmp_filtered/1(In1)
  Sum/1 -> OutputWithRamping/2, WithoutRamp/1
  RampUpOrDown/1 -> RampOutput/1, OutputWithRamping/1, SignalForSin_binary/1(In1)
  QuasiEnable/1 -> SignalForRamp_binary/1(In1)
  SignalForRamp_binary/1(Out1) -> RampUpOrDown/1
  Amplitude/1 -> PrescaledAmp/1
  signal with gain/1 -> Sum/1
  Frequency/1 -> ProductPhase/2
  SignalForSin_binary/1(Out1) -> ProductPhase/1
  ProductPhase/1 -> Subsystem/2(In2)
  AveragedOffset_filtered/1(Out1) -> Sum/2, OffsetOutput/1
  PrescaledOffset/1 -> AveragedOffset_filtered/1(In1)
  PreGain/1 -> PrescaledAmp/2, PrescaledOffset/2
  OutputWithRamping/1 -> SignalOutput/1
  AveragedAmp_filtered/1(Out1) -> signal with gain/2, AmplitudeOutput/1
  Sum1/1 -> PrescaledOffset/1
  Offset/1 -> Sum1/1
  PitchBias/1 -> Sum1/2
  AveragedTau_filtered/1(Out1) -> Subsystem/1(split cycle mu)
  split cycle mu/1 -> AveragedTau_filtered/1(In1)
  Subsystem/1(split cycle signal) -> signal with gain/1

== system opti_debug/Signal generater/signal generator1/SignalSaturationLimit ==
  BiasMax : Inport
  SignalRaw : Inport  Port=2
  GainBias : Gain
  MaxOf : MinMax  Function=max  Inputs=2
  MinOf : MinMax  Inputs=2
  ground : Constant
  SignalSatd : Outport
  wires:
  BiasMax/1 -> GainBias/1
  SignalRaw/1 -> MinOf/2
  MinOf/1 -> MaxOf/1
  MaxOf/1 -> SignalSatd/1
  GainBias/1 -> MinOf/1
  ground/1 -> MaxOf/2

== system opti_debug/Signal generater/signal generator1/SignalSaturationLimit1 ==
  BiasMax : Inport
  SignalRaw : Inport  Port=2
  GainBias : Gain
  MaxOf : MinMax  Function=max  Inputs=2
  MinOf : MinMax  Inputs=2
  ground : Constant
  SignalSatd : Outport
  wires:
  BiasMax/1 -> GainBias/1
  SignalRaw/1 -> MinOf/2
  MinOf/1 -> MaxOf/1
  MaxOf/1 -> SignalSatd/1
  GainBias/1 -> MinOf/1
  ground/1 -> MaxOf/2

== system opti_debug/Signal generater/signal generator1/SignalSaturationLimit2 ==
  BiasMax : Inport
  SignalRaw : Inport  Port=2
  GainBias : Gain
  MaxOf : MinMax  Function=max  Inputs=2
  MinOf : MinMax  Inputs=2
  ground : Constant
  SignalSatd : Outport
  wires:
  BiasMax/1 -> GainBias/1
  SignalRaw/1 -> MinOf/2
  MinOf/1 -> MaxOf/1
  MaxOf/1 -> SignalSatd/1
  GainBias/1 -> MinOf/1
  ground/1 -> MaxOf/2

== system opti_debug/Signal generater/signal generator1/SignalSaturationLimit3 ==
  BiasMax : Inport
  SignalRaw : Inport  Port=2
  GainBias : Gain
  MaxOf : MinMax  Function=max  Inputs=2
  MinOf : MinMax  Inputs=2
  ground : Constant
  SignalSatd : Outport
  wires:
  BiasMax/1 -> GainBias/1
  SignalRaw/1 -> MinOf/2
  MinOf/1 -> MaxOf/1
  MaxOf/1 -> SignalSatd/1
  GainBias/1 -> MinOf/1
  ground/1 -> MaxOf/2

== system opti_debug/Signal generater/signal generator1/signal generator 1 ==
  quasi enable : Inport
  max voltage : Inport  Port=2
  frequency : Inport  Port=3
  half amplitude : Inport  Port=4
  OutputWithRamping : Product  RndMeth=Zero
  RampUpOrDown : DiscreteIntegrator  gainval=1000  SampleTime=mdl.T_high  LimitOutput=on  UpperSaturationLimit=1  LowerSaturationLimit=0  ICPrevOutput=DiscIntNeverNeededParam  ICPrevScaledInput=DiscIntNeverNeededParam
  Scope1 : Scope  Commented=on
  Scope2 : Scope  Commented=on
  SignalForRamp_binary : Subsystem
  SignalSaturationLimit4 : Subsystem
  Terminator : Terminator
  deg to rad : Gain  Gain=pi/180
  get max voltage : Subsystem
  original sine wave : Subsystem
  phase offset : Constant  Value=180
  square root of sine wave : Subsystem
  SignalSatd : Outport
  wires:
  RampUpOrDown/1 -> OutputWithRamping/1
  max voltage/1 -> get max voltage/2(max voltage)
  quasi enable/1 -> Scope2/1, SignalForRamp_binary/1(EnableSignal), get max voltage/1(QuasiEnable)
  SignalForRamp_binary/1(Out1) -> RampUpOrDown/1
  phase offset/1 -> deg to rad/1
  OutputWithRamping/1 -> SignalSaturationLimit4/2(SignalRaw)
  get max voltage/1(max signa;) -> Scope1/1, SignalSaturationLimit4/1(Max)
  SignalSaturationLimit4/1(SignalSatd) -> SignalSatd/1
  frequency/1 -> original sine wave/2(In2), square root of sine wave/2(frequency)
  deg to rad/1 -> original sine wave/1(In1), square root of sine wave/1(phase)
  half amplitude/1 -> original sine wave/3(new_amplitude), square root of sine wave/3(half amplitude)
  square root of sine wave/1(Out1) -> OutputWithRamping/2
  original sine wave/1(Out1) -> Terminator/1

== system opti_debug/Signal generater/signal generator1/signal generator 2 ==
  quasi enable : Inport
  max voltage : Inport  Port=2
  frequency : Inport  Port=3
  half amplitude : Inport  Port=4
  2pi : Gain  Gain=2*pi
  Add1 : Sum
  Add2 : Sum
  Gain1 : Gain  Gain=-1
  OutputWithRamping : Product  RndMeth=Zero
  RampUpOrDown : DiscreteIntegrator  gainval=1000  SampleTime=mdl.T_high  LimitOutput=on  UpperSaturationLimit=1  LowerSaturationLimit=0  ICPrevOutput=DiscIntNeverNeededParam  ICPrevScaledInput=DiscIntNeverNeededParam
  SignalForRamp_binary : Subsystem
  SignalSaturationLimit4 : Subsystem
  Subsystem : Subsystem
  Terminator : Terminator
  deg to rad : Gain  Gain=pi/180
  first harmonic : Trigonometry  Operator=cos  OutputSignalType=real
  get max voltage : Subsystem
  omega*t : DiscreteIntegrator  SampleTime=-1  ICPrevOutput=DiscIntNeverNeededParam  ICPrevScaledInput=DiscIntNeverNeededParam
  phase offset : Constant  Value=0
  signal with gain1 : Product  RndMeth=Zero
  square root of sine wave : Subsystem
  SignalSatd : Outport
  wires:
  first harmonic/1 -> Gain1/1
  Subsystem/1(output) -> Add2/2, signal with gain1/2
  RampUpOrDown/1 -> OutputWithRamping/1
  deg to rad/1 -> square root of sine wave/1(phase), Add1/1
  Add1/1 -> first harmonic/1
  max voltage/1 -> get max voltage/2(max voltage)
  2pi/1 -> omega*t/1
  signal with gain1/1 -> Add2/1
  omega*t/1 -> Add1/2
  Gain1/1 -> Subsystem/1(cos wave), signal with gain1/1
  quasi enable/1 -> SignalForRamp_binary/1(EnableSignal), get max voltage/1(QuasiEnable)
  SignalForRamp_binary/1(Out1) -> RampUpOrDown/1
  phase offset/1 -> deg to rad/1
  OutputWithRamping/1 -> SignalSaturationLimit4/2(SignalRaw)
  get max voltage/1(max signa;) -> SignalSaturationLimit4/1(Max)
  SignalSaturationLimit4/1(SignalSatd) -> SignalSatd/1
  half amplitude/1 -> square root of sine wave/3(half amplitude), Subsystem/2(new_amplitude)
  frequency/1 -> square root of sine wave/2(frequency), 2pi/1
  Add2/1 -> Terminator/1
  square root of sine wave/1(Out1) -> OutputWithRamping/2

== system opti_debug/Signal generater/signal generator1/signal generator 3 ==
  quasi enable : Inport
  max voltage : Inport  Port=2
  frequency : Inport  Port=3
  half amplitude : Inport  Port=4
  2pi : Gain  Gain=2*pi
  Add1 : Sum
  Add2 : Sum
  Gain1 : Gain  Gain=-1
  OutputWithRamping : Product  RndMeth=Zero
  RampUpOrDown : DiscreteIntegrator  gainval=1000  SampleTime=mdl.T_high  LimitOutput=on  UpperSaturationLimit=1  LowerSaturationLimit=0  ICPrevOutput=DiscIntNeverNeededParam  ICPrevScaledInput=DiscIntNeverNeededParam
  SignalForRamp_binary : Subsystem
  SignalSaturationLimit4 : Subsystem
  Subsystem : Subsystem
  Terminator : Terminator
  deg to rad : Gain  Gain=pi/180
  first harmonic : Trigonometry  Operator=cos  OutputSignalType=real
  get max voltage : Subsystem
  omega*t : DiscreteIntegrator  SampleTime=-1  ICPrevOutput=DiscIntNeverNeededParam  ICPrevScaledInput=DiscIntNeverNeededParam
  phase offset : Constant  Value=180
  signal with gain1 : Product  RndMeth=Zero
  square root of sine wave : Subsystem
  SignalSatd : Outport
  wires:
  first harmonic/1 -> Gain1/1
  RampUpOrDown/1 -> OutputWithRamping/1
  deg to rad/1 -> square root of sine wave/1(phase), Add1/1
  Add1/1 -> first harmonic/1
  max voltage/1 -> get max voltage/2(max voltage)
  2pi/1 -> omega*t/1
  signal with gain1/1 -> Add2/1
  omega*t/1 -> Add1/2
  Gain1/1 -> Subsystem/1(cos wave), signal with gain1/1
  quasi enable/1 -> SignalForRamp_binary/1(EnableSignal), get max voltage/1(QuasiEnable)
  SignalForRamp_binary/1(Out1) -> RampUpOrDown/1
  phase offset/1 -> deg to rad/1
  OutputWithRamping/1 -> SignalSaturationLimit4/2(SignalRaw)
  get max voltage/1(max signa;) -> SignalSaturationLimit4/1(Max)
  SignalSaturationLimit4/1(SignalSatd) -> SignalSatd/1
  frequency/1 -> square root of sine wave/2(frequency), 2pi/1
  half amplitude/1 -> square root of sine wave/3(half amplitude), Subsystem/2(new_amplitude)
  Subsystem/1(output) -> Add2/2, signal with gain1/2
  Add2/1 -> Terminator/1
  square root of sine wave/1(Out1) -> OutputWithRamping/2

== system opti_debug/Signal generater/signal generator1/signal generator 4 ==
  quasi enable : Inport
  max voltage : Inport  Port=2
  frequency : Inport  Port=3
  half amplitude : Inport  Port=4
  2pi : Gain  Gain=2*pi
  Add1 : Sum
  Add2 : Sum
  Gain1 : Gain  Gain=-1
  OutputWithRamping : Product  RndMeth=Zero
  RampUpOrDown : DiscreteIntegrator  gainval=1000  SampleTime=mdl.T_high  LimitOutput=on  UpperSaturationLimit=1  LowerSaturationLimit=0  ICPrevOutput=DiscIntNeverNeededParam  ICPrevScaledInput=DiscIntNeverNeededParam
  SignalForRamp_binary : Subsystem
  SignalSaturationLimit4 : Subsystem
  Subsystem : Subsystem
  Terminator : Terminator
  deg to rad : Gain  Gain=pi/180
  first harmonic : Trigonometry  Operator=cos  OutputSignalType=real
  get max voltage : Subsystem
  omega*t : DiscreteIntegrator  SampleTime=-1  ICPrevOutput=DiscIntNeverNeededParam  ICPrevScaledInput=DiscIntNeverNeededParam
  phase offset : Constant  Value=0
  signal with gain1 : Product  RndMeth=Zero
  square root of sine wave : Subsystem
  SignalSatd : Outport
  wires:
  first harmonic/1 -> Gain1/1
  RampUpOrDown/1 -> OutputWithRamping/1
  deg to rad/1 -> square root of sine wave/1(phase), Add1/1
  Add1/1 -> first harmonic/1
  max voltage/1 -> get max voltage/2(max voltage)
  2pi/1 -> omega*t/1
  signal with gain1/1 -> Add2/1
  omega*t/1 -> Add1/2
  Gain1/1 -> signal with gain1/1, Subsystem/1(cos wave)
  quasi enable/1 -> SignalForRamp_binary/1(EnableSignal), get max voltage/1(QuasiEnable)
  SignalForRamp_binary/1(Out1) -> RampUpOrDown/1
  phase offset/1 -> deg to rad/1
  OutputWithRamping/1 -> SignalSaturationLimit4/2(SignalRaw)
  get max voltage/1(max signa;) -> SignalSaturationLimit4/1(Max)
  SignalSaturationLimit4/1(SignalSatd) -> SignalSatd/1
  half amplitude/1 -> square root of sine wave/3(half amplitude), Subsystem/2(new_amplitude)
  frequency/1 -> square root of sine wave/2(frequency), 2pi/1
  Subsystem/1(output) -> signal with gain1/2, Add2/2
  Add2/1 -> Terminator/1
  square root of sine wave/1(Out1) -> OutputWithRamping/2
